simulink library "SigiLib"  (R2025b)
settings: Solver=VariableStepAuto  StartTime=0.0  StopTime=10.0  RelTol=1e-3
undefined symbols (not defined in the file): fractalcoef, X, Y, Z
libraries: sm_lib x47, nesl_utility x13, simulink x9, fl_lib x6, raspberrypiCommlib x5, $bdroot x4, ee_lib x3, mspsensorlib x1, slpidlib x1
(part 1 of 2)
settings Model: Creator=vlenzi  LastModifiedBy=resjoehr
settings RTWCC: GPUComputeCapability=3.5

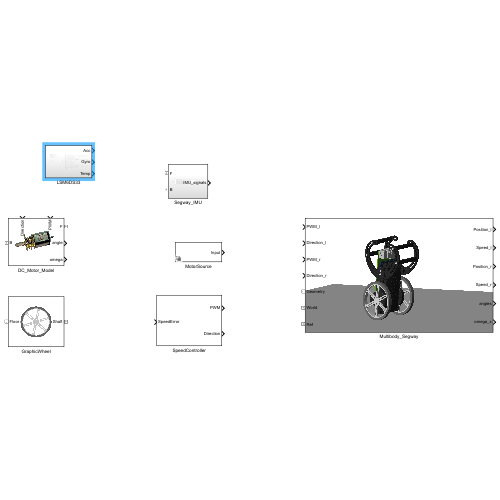
[thumbnail: Simulink's stored preview of the top-level diagram]
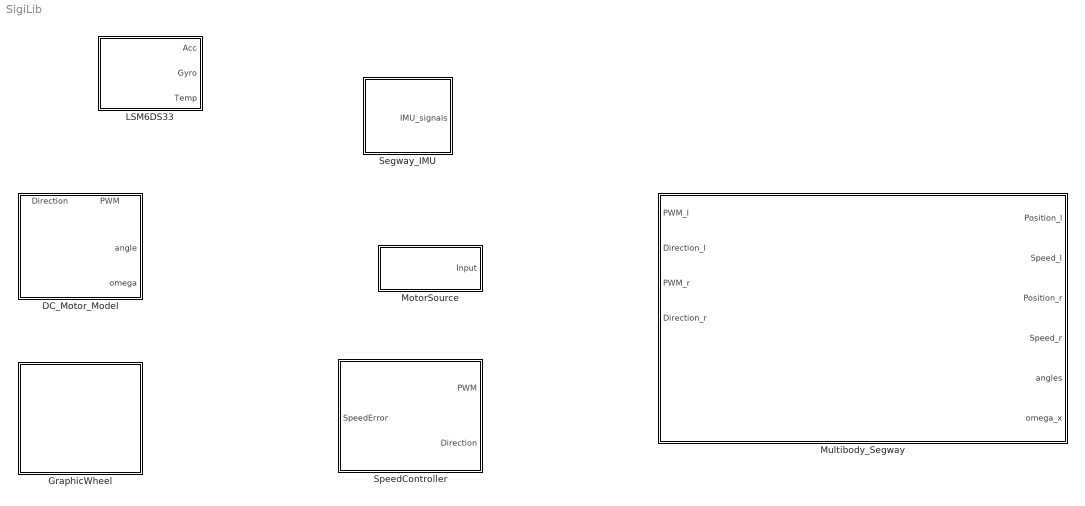
== system SigiLib ==
  DC_Motor_Model : Subsystem  mask{arm_induct=0, nlspeed=0, stall_T=0, rotor_I=0, rotor_damp=0, gear_ratio=0}
      mask prompts: arm_induct "Arm Inductance"; nlspeed "No Load Speed"; stall_T "Stall Torque"; rotor_I "Rotor Inertia"; rotor_damp "Rotor Damping"; gear_ratio "Gear Ratio (external gear box)"
      settings: PortSchema="{\"entries\":[{\"content\":{\"sides\":[{\"content\":{\"connectorIds\":[\"LConn1\"]},\"type\":\"ConnectorPlacement.EquallySpacedRectSide\",\"uuid\":\"0f359635-e508-4ae0-888d-e7a4bdac0ad6\"},{\"content\":{\"connectorIds\":[\"RConn1\",\"Out1\",\"Out2\"],\"side\":\"RIGHT\"},\"type\":\"ConnectorPlacement.EquallySpacedRectSide\",\"uuid\":\"bdc1407e-b686-4053-bd54-ae80f62d25cc\"},{\"content\":{\"connectorIds\":[\"In1\",\"In2\"],\"side\":\"TOP\"},\"type\":\"ConnectorPlacement.EquallySpacedRectSide\",\"uuid\":\"c3ebbcbf-819a-4495-8528-c62fc3c649d7\"}]},\"type\":\"ConnectorPlacement.EquallySpacedConnector\",\"uuid\":\"e7614881-2b96-4b82-8f72-d1d459cee471\"}],\"packageUris\":[\"http://schema.mathworks.com/mf0/Connector/R2020b\"],\"version\":\"1.0\"}"
      mask DialogControl Control2 Prompt: Motor parameters:
      mask DialogControl Control1 Prompt: Please specify the motor parameters. Please note, they can typically be found in the specsheet.
      mask Display: image('DC_motor.jpg');
  GraphicWheel : Subsystem
      mask Display: image('wheel.jpg', [15,15,15,15,100,100]);
  LSM6DS33 : Subsystem
  MotorSource : Subsystem  Variant=on  VariantControlMode=label  LabelModeActiveChoice=Square  mask{amp=0}
      mask prompts: amp "Amplitude"
  Multibody_Segway : Subsystem  mask{Parameter3=0, Parameter2=0}
      mask prompts: Parameter3 "Motor right"; Parameter2 "Motor left"
      mask DialogControl Container1 Prompt: Description
      mask DialogControl Control1 Prompt: This block implements the physics of the Segway using Simscape Multibody
      mask DialogControl Container2 Prompt: Parameters
      mask Display: image('whole_sigi.jpg');
  Segway_IMU : Subsystem
  SpeedController : Subsystem  mask{p_gain=0, i_gain=0, d_gain=0, n_filter=0, direction=0}
      mask prompts: p_gain "P-Gain"; i_gain "I-Gain"; d_gain "D-Gain"; n_filter "Filter"

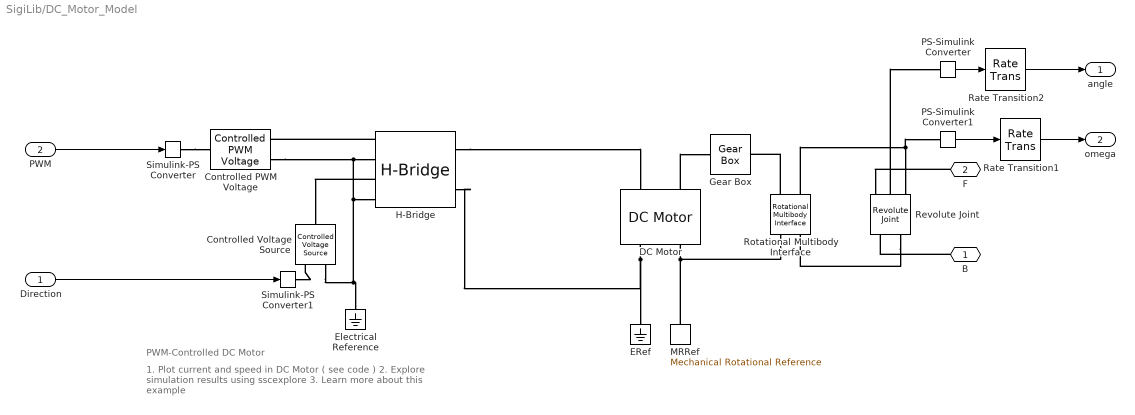
== system SigiLib/DC_Motor_Model ==
  note: PWM-Controlled DC Motor
  note: 1. Plot current and speed in DC Motor ( see code )
      | 2. Explore simulation results using sscexplore
      | 3. Learn more about this example
  Direction : Inport
  PWM : Inport  Port=2
  Controlled PWM Voltage : ee_lib/Integrated Circuits/Controlled PWM Voltage  F=1000 Hz  TD=0 s  pulse_width_offset=0 s  pulse_min=0 s  pwm_or_av=ee.enum.pwm_or_av.averaged  event_type=1  sample_time=5e-6 s  Vmin=0 V  Vmax=5 V  Vm=5 V  u_min=0  u_max=255
      settings: InternalSimscapePortConfiguration="{\"Bottom\":[],\"Left\":[{\"id\":\"u\",\"label\":\"u\",\"type\":\"input\"}],\"Right\":[{\"id\":\"p2\",\"label\":\"PWM\",\"type\":\"foundation.electrical.electrical\"},{\"id\":\"n2\",\"label\":\"REF\",\"type\":\"foundation.electrical.electrical\"}],\"Top\":[]}"
  Controlled Voltage Source : fl_lib/Electrical/Electrical Sources/Controlled Voltage Source
  DC Motor : ee_lib/Electromechanical/Brushed Motors/DC Motor  field_option=ee.enum.field_option.pm  Rf=100 Ohm  Lf=1 H  Laf=0.15 H  If0=0 A  parameterization=ee.enum.dcparam_option.torque_speed  Ra=3.38 Ohm  La=arm_induct H  emf_or_torque=ee.enum.emf_or_torque.kv  Kv=0.029 V/(rad/s)  Ki=6.876e-04 N*m/A  T_stall=stall_T N*m  w_max=nlspeed rpm  w_rated=2500 rpm  P_rated=10 W  V_rated=6 V  lam_param=ee.enum.lam_param.damping  i_noload=0 A  V_i_noload=1.5 V  J=rotor_I kg*m^2  lam=rotor_damp N*m/(rad/s)  speed0=0 rpm  alpha=3.93e-3 1/K  Tmeas=25 degC  thermal_mass=100 J/K  initial_temperature=25 degC
  ERef : fl_lib/Electrical/Electrical Elements/Electrical Reference
  Electrical Reference : fl_lib/Electrical/Electrical Elements/Electrical Reference
  Gear Box : fl_lib/Mechanical/Mechanisms/Gear Box  ratio=gear_ratio  t_in_specify=off  t_in_priority=None  t_in=0 N*m  t_in_nominal_specify=off  t_in_nominal_value=1  t_in_nominal_unit=N*m  t_out_specify=off  t_out_priority=None  t_out=0 N*m  t_out_nominal_specify=off  t_out_nominal_value=1  t_out_nominal_unit=N*m
  H-Bridge : ee_lib/Semiconductors & Converters/Converters/H-Bridge  supply_ports=ee.enum.supply_ports.hidesupply  pwm_or_av=ee.enum.pwm_or_av.averaged  regenerative_braking_mode=ee.enum.converters.regenerative_braking_mode.always_enabled  discontinuous=ee.enum.current_profile.continuous  freewheeling_mode=ee.enum.converters.freewheeling_mode.one_switch_one_diode  Rload=3.38+0.1 Ohm  Lload=1e-5 H  F=4 kHz  Venable=2.5 V  Vmax=5 V  Vreverse=.5 V  Vbrake=2.5 V  Vm=5 V  Ron=0.1 Ohm  Don=0.1 Ohm  Goff=1e-6 S  Tmeas=298.15 K  Ron2=0.1 Ohm  Don2=0.05 Ohm  Tmeas2=398.15 K  thermal_mass=100 J/K  initial_temperature=298.15 K
  MRRef : fl_lib/Mechanical/Rotational Elements/Mechanical Rotational Reference
  PS-Simulink Converter : nesl_utility/PS-Simulink Converter  PhysicalDomain=network_engine_domain  SubClassName=ps_output  LeftPortType=input  RightPortType=output  PseudoPeriodic=off  Frequencies=[]  VectorFormat=inherit  Unit=inherit  AffineConversion=off
  PS-Simulink Converter1 : nesl_utility/PS-Simulink Converter  PhysicalDomain=network_engine_domain  SubClassName=ps_output  LeftPortType=input  RightPortType=output  PseudoPeriodic=off  Frequencies=[]  VectorFormat=inherit  Unit=inherit  AffineConversion=off
  Rate Transition1 : RateTransition  OutPortSampleTime=0.01
  Rate Transition2 : RateTransition  OutPortSampleTime=0.01
  Revolute Joint : sm_lib/Joints/Revolute Joint  JointMode=Normal  CompositeWrenchDir=FollowerOnBase  CompositeWrenchFrame=BaseFrame  SenseConstraintForce=off  SenseConstraintTorque=off  SenseTotalForce=off  SenseTotalTorque=off  PositionTargetSpecify=off  PositionTargetPriority=High  PositionTargetValue=0  PositionTargetValueUnits=deg  VelocityTargetSpecify=off  VelocityTargetPriority=High  VelocityTargetValue=0  VelocityTargetValueUnits=deg/s  EquilibriumPosition=0  EquilibriumPositionUnits=deg  SpringStiffness=0  SpringStiffnessUnits=N*m/deg  DampingCoefficient=0  DampingCoefficientUnits=N*m/(deg/s)  LowerLimitSpecify=off  LowerLimitBound=-90  LowerLimitBoundUnits=deg  LowerLimitStiffness=1e4  LowerLimitStiffnessUnits=N*m/deg  LowerLimitDamping=10  LowerLimitDampingUnits=N*m/(deg/s)  LowerLimitTransitionRegionWidth=0.1  LowerLimitTransitionRegionWidthUnits=deg  UpperLimitSpecify=off  UpperLimitBound=90  UpperLimitBoundUnits=deg  UpperLimitStiffness=1e4  UpperLimitStiffnessUnits=N*m/deg  UpperLimitDamping=10  UpperLimitDampingUnits=N*m/(deg/s)  UpperLimitTransitionRegionWidth=0.1  UpperLimitTransitionRegionWidthUnits=deg  TorqueActuationMode=InputTorque  MotionActuationMode=ComputedMotion  SensePosition=on  SenseVelocity=on  SenseAcceleration=off  SenseTorqueForce=off  SenseLowerLimitTorqueForce=off  SenseUpperLimitTorqueForce=off
  Rotational Multibody Interface : fl_lib/Mechanical/Multibody Interfaces/Rotational Multibody Interface
  Simulink-PS Converter : nesl_utility/Simulink-PS Converter  PhysicalDomain=network_engine_domain  SubClassName=ps_input  LeftPortType=input  RightPortType=output  PseudoPeriodic=off  Frequencies=[]  NoiseDistribution=none  NoiseParameters=[]  Unit=1  AffineConversion=off  FilteringAndDerivatives=provide  SimscapeFilterOrder=1  InputFilterTimeConstant=0.001  UdotUserProvided=0
  Simulink-PS Converter1 : nesl_utility/Simulink-PS Converter  PhysicalDomain=network_engine_domain  SubClassName=ps_input  LeftPortType=input  RightPortType=output  PseudoPeriodic=off  Frequencies=[]  NoiseDistribution=none  NoiseParameters=[]  Unit=1  AffineConversion=off  FilteringAndDerivatives=provide  SimscapeFilterOrder=1  InputFilterTimeConstant=0.001  UdotUserProvided=0
  B : PMIOPort  Side=Left
  F : PMIOPort  Port=2  Side=Right
  angle : Outport
  omega : Outport  Port=2
  wires:
  PWM/1 -> Simulink-PS Converter/1
  Direction/1 -> Simulink-PS Converter1/1
  PS-Simulink Converter1/1 -> Rate Transition1/1
  PS-Simulink Converter/1 -> Rate Transition2/1
  Rate Transition2/1 -> angle/1
  Rate Transition1/1 -> omega/1
  connections:
  H-Bridge/RConn1 -- DC Motor/LConn1
  H-Bridge/LConn3 -- Controlled Voltage Source/LConn1
  Controlled Voltage Source/RConn2 -- Electrical Reference/LConn1 -- H-Bridge/LConn4 -- H-Bridge/LConn2 -- Controlled PWM Voltage/RConn2
  DC Motor/LConn2 -- Gear Box/LConn1
  MRRef/LConn1 -- Rotational Multibody Interface/LConn2 -- DC Motor/RConn2
  DC Motor/RConn1 -- ERef/LConn1 -- H-Bridge/RConn2
  H-Bridge/LConn1 -- Controlled PWM Voltage/RConn1
  Simulink-PS Converter/RConn1 -- Controlled PWM Voltage/LConn1
  Simulink-PS Converter1/RConn1 -- Controlled Voltage Source/RConn1
  Rotational Multibody Interface/RConn1 -- Revolute Joint/RConn3 -- PS-Simulink Converter1/LConn1
  Revolute Joint/LConn2 -- Rotational Multibody Interface/LConn1
  F/RConn1 -- Revolute Joint/RConn1
  B/RConn1 -- Revolute Joint/LConn1
  Rotational Multibody Interface/RConn2 -- Gear Box/RConn1
  Revolute Joint/RConn2 -- PS-Simulink Converter/LConn1

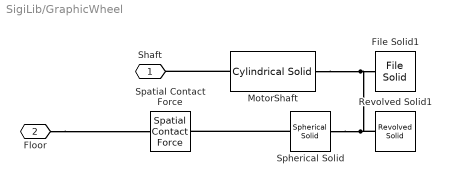
== system SigiLib/GraphicWheel ==
  File Solid1 : sm_lib/Body Elements/File Solid  ExtGeomFileName=Wheel.stl  UnitType=Custom  ExtGeomFileUnits=m  StepReaderType=HEX  ExportConvexHullGeometry=off  InertiaType=CalculateFromGeometry  BasedOnType=Density  Density=2000  DensityUnits=kg/m^3  Mass=1  MassUnits=kg  CenterOfMass=[0 0 0]  CenterOfMassUnits=m  MomentsOfInertia=[1 1 1]  MomentsOfInertiaUnits=kg*m^2  ProductsOfInertia=[0 0 0]  ProductsOfInertiaUnits=kg*m^2  GraphicType=FromGeometry  MarkerShape=Sphere  MarkerSize=10  GraphicVisPropType=SimpleVisualProperties  GraphicDiffuseColor=[1.0 1.0 1.0]  GraphicOpacity=1.0  GraphicSpecularColor=[0.5 0.5 0.5 1.0]  GraphicAmbientColor=[0.15 0.15 0.15 1.0]  GraphicEmissiveColor=[0.0 0.0 0.0 1.0]  GraphicShininess=75  DoExposeReferenceFrame=on  SerializedFrames=<Frames/>
  MotorShaft : sm_lib/Body Elements/Cylindrical Solid  CylinderRadius=1  CylinderRadiusUnits=mm  CylinderLength=10  CylinderLengthUnits=mm  ExportEntireGeometry=off  InertiaType=CalculateFromGeometry  BasedOnType=Density  Density=1000  DensityUnits=kg/m^3  Mass=1  MassUnits=kg  CenterOfMass=[0 0 0]  CenterOfMassUnits=m  MomentsOfInertia=[1 1 1]  MomentsOfInertiaUnits=kg*m^2  ProductsOfInertia=[0 0 0]  ProductsOfInertiaUnits=kg*m^2  GraphicType=FromGeometry  MarkerShape=Sphere  MarkerSize=10  GraphicVisPropType=SimpleVisualProperties  GraphicDiffuseColor=[0.5 0.5 0.5]  GraphicOpacity=1.0  GraphicSpecularColor=[0.5 0.5 0.5 1.0]  GraphicAmbientColor=[0.15 0.15 0.15 1.0]  GraphicEmissiveColor=[0.0 0.0 0.0 1.0]  GraphicShininess=75  DoExposeReferenceFrame=off  SerializedFrames=<Frames><Frame><Id>Frame1</Id><Value><Name>Bottom</Name><Origin><Source>GeometricFeature</Source><FeatureName>bottom surface</FeatureName></Origin><PrimaryAxis><DefinedDirection>+Z</DefinedDirection><Source>ReferenceFrame</Source><SourceDirection>+Z</SourceDirection><FeatureName></FeatureName></PrimaryAxis><SecondaryAxis><DefinedDirection>+X</DefinedDirection><Source>ReferenceFrame</Source><SourceDirection>+X</SourceDirection><FeatureName></FeatureName></SecondaryAxis></Value></Frame><Frame><Id>Frame2</Id><Value><Name>Top</Name><Origin><Source>GeometricFeature</Source><FeatureName>top surface</FeatureName></Origin><PrimaryAxis><DefinedDirection>+Z</DefinedDirection><Source>ReferenceFrame</Source><SourceDirection>+Z</SourceDirection><FeatureName></FeatureName></PrimaryAxis><SecondaryAxis><DefinedDirection>+X</DefinedDirection><Source>ReferenceFrame</Source><SourceDirection>+X</SourceDirection><FeatureName></FeatureName></SecondaryAxis></Value></Frame></Frames>
  Revolved Solid1 : sm_lib/Body Elements/Revolved Solid  RevolutionCrossSection=[3.5 0.5; 3.5 -0.5; 4 -0.5; 4 0.5]  RevolutionCrossSectionUnits=cm  RevolutionExtent=Full  RevolutionAngle=180  RevolutionAngleUnits=deg  ExportConvexHullGeometry=off  InertiaType=CalculateFromGeometry  BasedOnType=Density  Density=0  DensityUnits=kg/m^3  Mass=1  MassUnits=kg  CenterOfMass=[0 0 0]  CenterOfMassUnits=m  MomentsOfInertia=[1 1 1]  MomentsOfInertiaUnits=kg*m^2  ProductsOfInertia=[0 0 0]  ProductsOfInertiaUnits=kg*m^2  GraphicType=FromGeometry  MarkerShape=Sphere  MarkerSize=10  GraphicVisPropType=SimpleVisualProperties  GraphicDiffuseColor=[0.5 0.5 0.5]  GraphicOpacity=1.0  GraphicSpecularColor=[0.5 0.5 0.5 1.0]  GraphicAmbientColor=[0.15 0.15 0.15 1.0]  GraphicEmissiveColor=[0.0 0.0 0.0 1.0]  GraphicShininess=75  DoExposeReferenceFrame=on  SerializedFrames=<Frames/>
  Spatial Contact Force : sm_lib/Forces and Torques/Spatial Contact Force  SenseSeparationDistance=off  NormalForceType=SmoothSpringDamper  NormalStiffness=1e6  NormalStiffnessUnits=N/m  NormalDamping=1e3  NormalDampingUnits=N/(m/s)  NormalTransitionRegionWidth=1e-4  NormalTransitionRegionWidthUnits=m  FrictionType=SmoothStickSlip  CoefficientOfStaticFriction=1  CoefficientOfDynamicFriction=0.7  FrictionalCriticalVelocity=0.001  FrictionalCriticalVelocityUnits=m/s  SenseContactSignal=off  SensePenetrationDepth=off  SenseNormalVelocity=off  SenseTangentialVelocity=off  SensingForceTorqueDirection=BaseOnFollower  SensingForceTorqueResolutionFrame=ContactFrame  SenseNormalForce=off  SenseNormalForceMagnitude=off  SenseNormalTorque=off  SenseFrictionalForce=off  SenseFrictionalForceMagnitude=off  SenseFrictionalTorque=off  SenseTotalForce=off  SenseTotalTorque=off  SenseContactBaseRotation=off  SenseContactBaseTranslation=off  SenseContactFollowerRotation=off  SenseContactFollowerTranslation=off  ZeroCrossDetectContactStartAndEnd=off
  Spherical Solid : sm_lib/Body Elements/Spherical Solid  SphereRadius=4.05  SphereRadiusUnits=cm  ExportEntireGeometry=on  InertiaType=CalculateFromGeometry  BasedOnType=Density  Density=0  DensityUnits=kg/m^3  Mass=1  MassUnits=kg  CenterOfMass=[0 0 0]  CenterOfMassUnits=m  MomentsOfInertia=[1 1 1]  MomentsOfInertiaUnits=kg*m^2  ProductsOfInertia=[0 0 0]  ProductsOfInertiaUnits=kg*m^2  GraphicType=FromGeometry  MarkerShape=Sphere  MarkerSize=10  GraphicVisPropType=SimpleVisualProperties  GraphicDiffuseColor=[0.6 0 0]  GraphicOpacity=0.1  GraphicSpecularColor=[0.5 0.5 0.5 1.0]  GraphicAmbientColor=[0.15 0.15 0.15 1.0]  GraphicEmissiveColor=[0.0 0.0 0.0 1.0]  GraphicShininess=75  DoExposeReferenceFrame=on  SerializedFrames=<Frames/>
  Shaft : PMIOPort  Side=Right
  Floor : PMIOPort  Port=2  Side=Left
  connections:
  File Solid1/RConn1 -- MotorShaft/RConn1 -- Spherical Solid/RConn1 -- Revolved Solid1/RConn1
  Floor/RConn1 -- Spatial Contact Force/RConn1
  MotorShaft/LConn1 -- Shaft/RConn1
  Spherical Solid/LConn1 -- Spatial Contact Force/LConn1

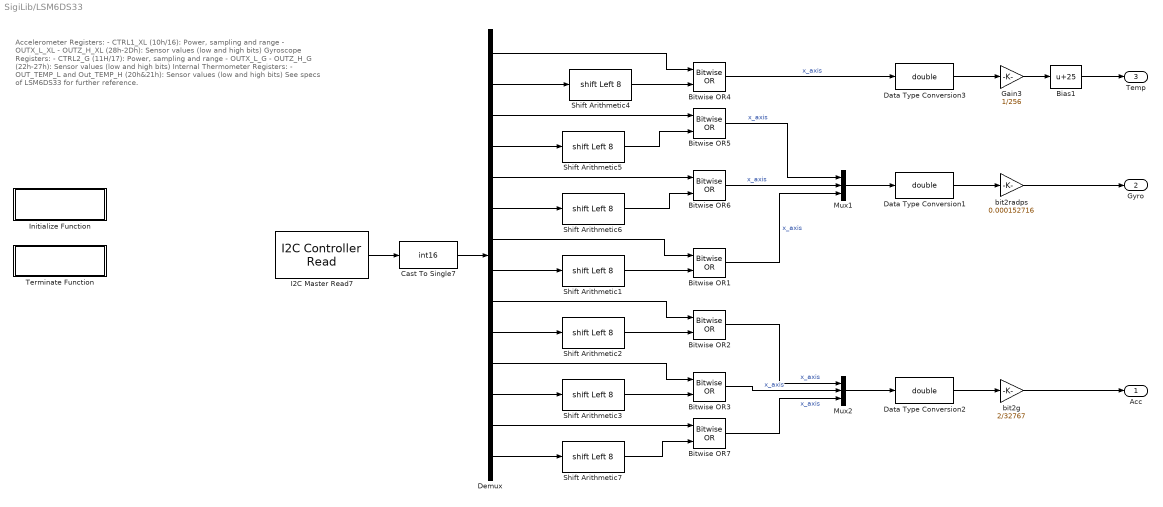
== system SigiLib/LSM6DS33 ==
  note: Accelerometer Registers:
      | - CTRL1_XL (10h/16): Power, sampling and range
      | - OUTX_L_XL - OUTZ_H_XL (28h-2Dh): Sensor values (low and high bits)
      |
      | Gyroscope Registers:
      | - CTRL2_G (11H/17): Power, sampling and range
      | - OUTX_L_G - OUTZ_H_G (22h-27h): Sensor values (low and high bits)
      |
      | Internal Thermometer Registers:
      | - OUT_TEMP_L and Out_TEMP_H (20h&21h): Sensor values (low and high bits)
      |
      | See specs of LSM6DS33 for further reference.
  Bias1 : Bias  Bias=25  SaturateOnIntegerOverflow=off
  Bitwise OR{1..7} (7 alike) : simulink/Logic and Bit Operations/Bitwise Operator  logicop=OR  UseBitMask=off  NumInputPorts=2  BitMask=bin2dec('11011001')  BitMaskRealWorld=Stored Integer
  Cast To Single7 : DataTypeConversion  OutDataTypeStr=int16  SaturateOnIntegerOverflow=off  RndMeth=Floor
  Data Type Conversion1 : DataTypeConversion  OutDataTypeStr=double  SaturateOnIntegerOverflow=off  RndMeth=Floor
  Data Type Conversion2 : DataTypeConversion  OutDataTypeStr=double  SaturateOnIntegerOverflow=off  RndMeth=Floor
  Data Type Conversion3 : DataTypeConversion  OutDataTypeStr=double  SaturateOnIntegerOverflow=off  RndMeth=Floor
  Demux : Demux  Outputs=14
  Gain3 : Gain  Gain=1/256
  I2C Master Read7 : raspberrypiCommlib/I2C Controller Read  BoardProperty=Pi 3 Model B+  I2CModule=1  Mode=Master  SlaveAddress=107  SlaveByteOrder=BigEndian  Direction=Receiver  RegisterAddressMode=on  RegisterAddress=hex2dec('20')  SlaveDataType=uint8  DataLength=14  NoAck=off  RepeatedStart=off  OutputStatus=off  SampleTime=0.01
  Initialize Function : Subsystem  TreatAsAtomicUnit=on
  Mux1 : Mux  Inputs=3
  Mux2 : Mux  Inputs=3
  Shift Arithmetic{1..7} (7 alike) : ArithShift  BitShiftNumber=8  BitShiftDirection=Left
  Terminate Function : Subsystem  TreatAsAtomicUnit=on
  bit2g : Gain  Gain=2/32767
  bit2radps : Gain  Gain=0.000152716
  Acc : Outport  Unit=g
  Gyro : Outport  Port=2  Unit=rad/s
  Temp : Outport  Port=3
  wires:
  Cast To Single7/1 -> Demux/1
  Shift Arithmetic4/1 -> Bitwise OR4/2
  Bitwise OR4/1 -> Data Type Conversion3/1  "x_axis"
  Shift Arithmetic6/1 -> Bitwise OR6/2
  Demux/1 -> Bitwise OR4/1
  Mux1/1 -> Data Type Conversion1/1
  Demux/5 -> Bitwise OR6/1
  Demux/6 -> Shift Arithmetic6/1
  I2C Master Read7/1 -> Cast To Single7/1
  Bitwise OR6/1 -> Mux1/2  "x_axis"
  Demux/4 -> Shift Arithmetic5/1
  Shift Arithmetic5/1 -> Bitwise OR5/2
  Demux/3 -> Bitwise OR5/1
  Demux/2 -> Shift Arithmetic4/1
  Bitwise OR5/1 -> Mux1/1  "x_axis"
  Data Type Conversion1/1 -> bit2radps/1
  Shift Arithmetic3/1 -> Bitwise OR3/2
  Bitwise OR3/1 -> Mux2/2  "x_axis"
  Bitwise OR1/1 -> Mux1/3  "x_axis"
  Shift Arithmetic1/1 -> Bitwise OR1/2
  Demux/7 -> Bitwise OR1/1
  Mux2/1 -> Data Type Conversion2/1
  Bitwise OR2/1 -> Mux2/1  "x_axis"
  Shift Arithmetic2/1 -> Bitwise OR2/2
  Demux/9 -> Bitwise OR2/1
  Demux/10 -> Shift Arithmetic2/1
  Demux/8 -> Shift Arithmetic1/1
  Demux/11 -> Bitwise OR3/1
  Demux/12 -> Shift Arithmetic3/1
  Demux/13 -> Bitwise OR7/1
  Shift Arithmetic7/1 -> Bitwise OR7/2
  Demux/14 -> Shift Arithmetic7/1
  Bitwise OR7/1 -> Mux2/3  "x_axis"
  Data Type Conversion2/1 -> bit2g/1
  Gain3/1 -> Bias1/1
  Bias1/1 -> Temp/1
  Data Type Conversion3/1 -> Gain3/1
  bit2g/1 -> Acc/1
  bit2radps/1 -> Gyro/1

== system SigiLib/MotorSource ==
  note: 1) Add Subsystem or Model blocks as valid variant choices.
      | 2) You cannot connect blocks at this level. At simulation, connectivity is automatically
      | determined, based on the active variant and port name matching.
  Subsystem : Subsystem  VariantControl=Custom
  Subsystem1 : Subsystem  VariantControl=Square
  Subsystem2 : Subsystem  VariantControl=Ramp
  Input : Outport

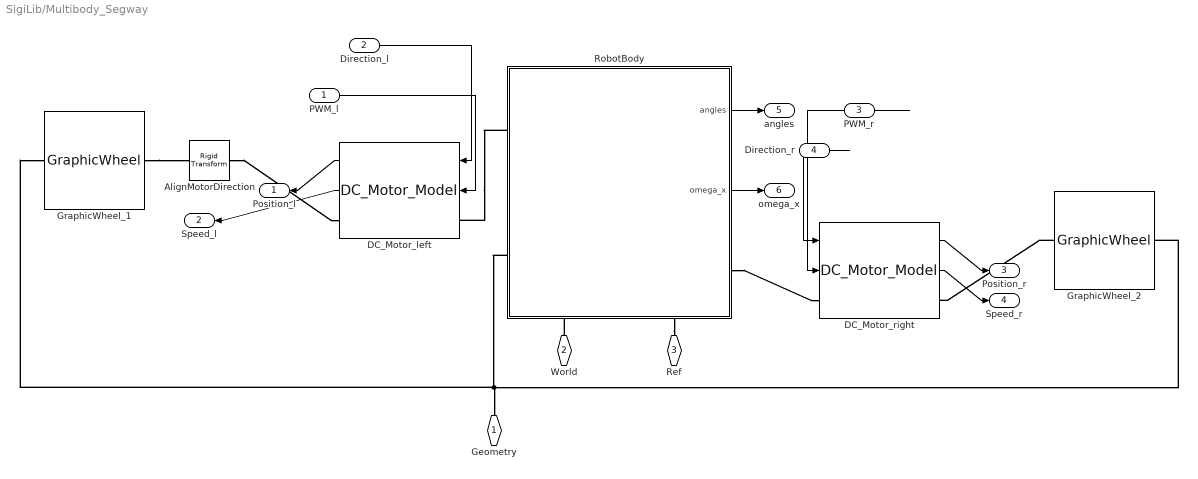
== system SigiLib/Multibody_Segway ==
  PWM_l : Inport
  Direction_l : Inport  Port=2
  PWM_r : Inport  Port=3
  Direction_r : Inport  Port=4
  AlignMotorDirection : sm_lib/Frames and Transforms/Rigid Transform  RotationMethod=StandardAxis  FollAlignAxisA=+Z  BaseAlignAxisA=-Z  FollAlignAxisB=+Y  BaseAlignAxisB=+Z  RotationStandardAxis=+Y  RotationAngle=180  RotationAngleUnits=deg  RotationArbitraryAxis=[0 0 1]  RotationSequenceAxes=FollowerAxes  RotationSequence=XYX  RotationSequenceAngles=[0 0 0]  RotationSequenceAnglesUnits=deg  RotationMatrix=[1 0 0; 0 1 0; 0 0 1]  Quaternion=[1 0 0 0]  TranslationMethod=None  TranslationCartesianOffset=[0 0 -0.014]  TranslationCartesianOffsetUnits=m  TranslationStandardAxis=+Z  TranslationStandardOffset=0  TranslationStandardOffsetUnits=m  TranslationROffset=0  TranslationROffsetUnits=m  TranslationThetaOffset=0  TranslationThetaOffsetUnits=deg  TranslationZOffset=0  TranslationZOffsetUnits=m
  DC_Motor_left : $bdroot/DC_Motor_Model  arm_induct=motor_left.arm_induct  nlspeed=motor_left.nlspeed  stall_T=motor_left.stall_T  rotor_I=motor_left.rotor_I  rotor_damp=motor_left.rotor_damp  gear_ratio=motor_left.gear_ratio
  DC_Motor_right : $bdroot/DC_Motor_Model  arm_induct=motor_right.arm_induct  nlspeed=motor_right.nlspeed  stall_T=motor_right.stall_T  rotor_I=motor_right.rotor_I  rotor_damp=motor_right.rotor_damp  gear_ratio=motor_right.gear_ratio
  GraphicWheel_1 : $bdroot/GraphicWheel  SystemSampleTime=-1  VariantActivationTime=update diagram  EmptyChoice=off  PassThrough=off  PassThroughVariantControl=(default)  EmptyChoiceVariantControl=(default)  AllowFlexibleInterface=on  Latency=0  AutoFrameSizeCalculation=off
      link override Spherical Solid: GraphicOpacity=0.4
  GraphicWheel_2 : $bdroot/GraphicWheel  SystemSampleTime=-1  VariantActivationTime=update diagram  EmptyChoice=off  PassThrough=off  PassThroughVariantControl=(default)  EmptyChoiceVariantControl=(default)  AllowFlexibleInterface=on  Latency=0  AutoFrameSizeCalculation=off
  RobotBody : Subsystem
      settings: PortSchema="{\"entries\":[{\"content\":{\"sides\":[{\"content\":{\"connectorIds\":[\"LConn1\",\"LConn2\"]},\"type\":\"ConnectorPlacement.EquallySpacedRectSide\",\"uuid\":\"3f35a83b-acf9-4542-85ca-c3be7738438d\"},{\"content\":{\"connectorIds\":[\"Out1\",\"Out2\",\"RConn1\"],\"side\":\"RIGHT\"},\"type\":\"ConnectorPlacement.EquallySpacedRectSide\",\"uuid\":\"c08ff41f-e4b1-40fb-853d-24ced0702649\"},{\"content\":{\"side\":\"TOP\"},\"type\":\"ConnectorPlacement.EquallySpacedRectSide\",\"uuid\":\"d298c9e2-1711-4257-8e5b-24fb1711ca30\"},{\"content\":{\"connectorIds\":[\"RConn2\",\"RConn3\"],\"side\":\"BOTTOM\"},\"type\":\"ConnectorPlacement.EquallySpacedRectSide\",\"uuid\":\"0a2d3d52-b6dd-493e-8124-2dc32b2e7700\"}]},\"type\":\"ConnectorPlacement.EquallySpacedConnector\",\"uuid\":\"2a993940-985c-47f0-a186-f410faa28ad3\"}],\"packageUris\":[\"http://schema.mathworks.com/mf0/Connector/R2020b\"],\"version\":\"1.0\"}"
      mask Display: image('sigi_body.jpg');
  Geometry : PMIOPort  Side=Left
  World : PMIOPort  Port=2  Side=Left
  Ref : PMIOPort  Port=3  Side=Left
  Position_l : Outport
  Speed_l : Outport  Port=2
  Position_r : Outport  Port=3
  Speed_r : Outport  Port=4
  angles : Outport  Port=5
  omega_x : Outport  Port=6
  wires:
  DC_Motor_right/2 -> Speed_r/1
  DC_Motor_left/2 -> Speed_l/1
  DC_Motor_right/1 -> Position_r/1
  PWM_r/1 -> DC_Motor_right/2
  Direction_r/1 -> DC_Motor_right/1
  RobotBody/2(omega_x) -> omega_x/1
  RobotBody/1(angles) -> angles/1
  DC_Motor_left/1 -> Position_l/1
  Direction_l/1 -> DC_Motor_left/1
  PWM_l/1 -> DC_Motor_left/2
  connections:
  RobotBody/LConn1 -- DC_Motor_left/LConn1
  AlignMotorDirection/LConn1 -- DC_Motor_left/RConn1
  RobotBody/RConn1 -- DC_Motor_right/LConn1
  GraphicWheel_1/RConn1 -- AlignMotorDirection/RConn1
  RobotBody/LConn2 -- GraphicWheel_1/LConn1 -- GraphicWheel_2/LConn1 -- Geometry/RConn1
  World/RConn1 -- RobotBody/RConn2
  GraphicWheel_2/RConn1 -- DC_Motor_right/RConn1
  RobotBody/RConn3 -- Ref/RConn1

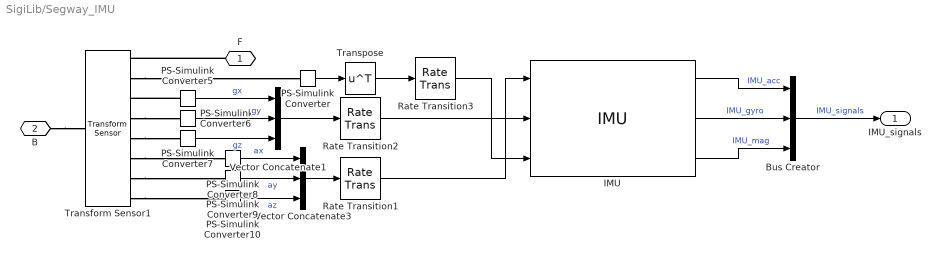
== system SigiLib/Segway_IMU ==
  Bus Creator : BusCreator  Inputs=3  OutDataTypeStr=Bus: IMU_signals
      settings: InheritFromInputs=off
  IMU : mspsensorlib/IMU  DispRefFrame=NED  TemperaturePort=off  Temperature=25  MagneticFieldPort=off  MagneticFieldNED=[ 27.5550, -2.4169, -16.0849 ]  MagneticFieldENU=[ -2.4169, 27.5550, 16.0849 ]  SeedDouble=67  SimulateUsing=Interpreted execution  AccelParamsMeasurementRange=19.62  AccelParamsResolution=5.9841e-4  AccelParamsConstantBias=[ 0, 0, 0 ]  AccelParamsAxesMisalignment=[ 100, 0, 0; 0, 100, 0; 0, 0, 100 ]  AccelParamsNoiseDensity=[ 0.1213e-3, 0.1072e-3, 0.2141e-3 ]  AccelParamsBiasInstability=[ 0.0402e-3, 0.0923e-3, 0.137e-3 ]  AccelParamsBiasInstabilityNumerator=fractalcoef().Numerator  AccelParamsBiasInstabilityDenominator=fractalcoef().Denominator  AccelParamsRandomWalk=[ 0.0399e-4, 0.1093e-4, 0.3611e-4 ]  AccelParamsNoiseType=double-sided  AccelParamsTemperatureBias=[ 0, 0, 0 ]  AccelParamsTemperatureScaleFactor=[ 0, 0, 0 ]  GyroParamsMeasurementRange=245  GyroParamsResolution=0.00875  GyroParamsConstantBias=[ 0.0527, -0.1277, -0.0283 ]  GyroParamsAxesMisalignment=[ 100, 0, 0; 0, 100, 0; 0, 0, 100 ]  GyroParamsAccelerationBias=[ 0, 0, 0 ]  GyroParamsNoiseDensity=[ 0.0034, 0.0046, 0.0016 ]  GyroParamsBiasInstability=[ 0.0006069, 0.0009649, 0.0004479 ]  GyroParamsBiasInstabilityNumerator=fractalcoef().Numerator  GyroParamsBiasInstabilityDenominator=fractalcoef().Denominator  GyroParamsRandomWalk=[ 0.00005272, 0.00007008, 0.00005776 ]  GyroParamsNoiseType=double-sided  GyroParamsTemperatureBias=[ 0, 0, 0 ]  GyroParamsTemperatureScaleFactor=[ 0, 0, 0 ]  MagParamsMeasurementRange=Inf  MagParamsResolution=0  MagParamsConstantBias=[ 0, 0, 0 ]  MagParamsAxesMisalignment=[ 100, 0, 0; 0, 100, 0; 0, 0, 100 ]  MagParamsNoiseDensity=[ 0, 0, 0 ]  MagParamsBiasInstability=[ 0, 0, 0 ]  MagParamsBiasInstabilityNumerator=fractalcoef().Numerator  MagParamsBiasInstabilityDenominator=fractalcoef().Denominator  MagParamsRandomWalk=[ 0, 0, 0 ]  MagParamsNoiseType=double-sided  MagParamsTemperatureBias=[ 0, 0, 0 ]  MagParamsTemperatureScaleFactor=[ 0, 0, 0 ]
  PS-Simulink Converter{,5..10} (7 alike) : nesl_utility/PS-Simulink Converter  PhysicalDomain=network_engine_domain  SubClassName=ps_output  LeftPortType=input  RightPortType=output  PseudoPeriodic=off  Frequencies=[]  VectorFormat=inherit  Unit=inherit  AffineConversion=off
  Rate Transition1 : RateTransition  OutPortSampleTime=0.01
  Rate Transition2 : RateTransition  OutPortSampleTime=0.01
  Rate Transition3 : RateTransition  OutPortSampleTime=0.01
  Transform Sensor1 : sm_lib/Frames and Transforms/Transform Sensor  MeasurementFrame=World  RotationSequence=XYX  SenseAngle=off  SenseAxis=off  SenseQ=on  SenseR=off  SenseRotationSequence=off  SenseOmegaX=on  SenseOmegaY=on  SenseOmegaZ=on  SenseOmega=off  SenseQDot=off  SenseRDot=off  SenseRotationSequenceDot=off  SenseAlphaX=off  SenseAlphaY=off  SenseAlphaZ=off  SenseAlpha=off  SenseQDDot=off  SenseRDDot=off  SenseX=off  SenseY=off  SenseZ=off  SenseXYZ=off  SenseRad=off  SenseAzim=off  SenseDist=off  SenseInc=off  SenseXDot=off  SenseYDot=off  SenseZDot=off  SenseXYZDot=off  SenseRadDot=off  SenseAzimDot=off  SenseDistDot=off  SenseIncDot=off  SenseXDDot=on  SenseYDDot=on  SenseZDDot=on  SenseXYZDDot=off  SenseRadDDot=off  SenseAzimDDot=off  SenseDistDDot=off  SenseIncDDot=off
  Transpose : Math  Operator=transpose
  Vector Concatenate1 : Concatenate  NumInputs=3  Mode=Multidimensional array  ConcatenateDimension=2
  Vector Concatenate3 : Concatenate  NumInputs=3  Mode=Multidimensional array  ConcatenateDimension=2
  F : PMIOPort  Side=Left
  B : PMIOPort  Port=2  Side=Left
  IMU_signals : Outport
  wires:
  PS-Simulink Converter5/1 -> Vector Concatenate1/1  "gx"
  PS-Simulink Converter6/1 -> Vector Concatenate1/2  "gy"
  PS-Simulink Converter7/1 -> Vector Concatenate1/3  "gz"
  PS-Simulink Converter8/1 -> Vector Concatenate3/1  "ax"
  PS-Simulink Converter9/1 -> Vector Concatenate3/2  "ay"
  PS-Simulink Converter10/1 -> Vector Concatenate3/3  "az"
  Vector Concatenate1/1 -> Rate Transition2/1
  Vector Concatenate3/1 -> Rate Transition1/1
  PS-Simulink Converter/1 -> Transpose/1
  Transpose/1 -> Rate Transition3/1
  IMU/1 -> Bus Creator/1  "IMU_acc"
  IMU/2 -> Bus Creator/2  "IMU_gyro"
  Rate Transition1/1 -> IMU/1
  Rate Transition2/1 -> IMU/2
  Rate Transition3/1 -> IMU/3
  IMU/3 -> Bus Creator/3  "IMU_mag"
  Bus Creator/1 -> IMU_signals/1  "IMU_signals"
  connections:
  F/RConn1 -- Transform Sensor1/RConn1
  B/RConn1 -- Transform Sensor1/LConn1
  PS-Simulink Converter5/LConn1 -- Transform Sensor1/RConn3
  Transform Sensor1/RConn4 -- PS-Simulink Converter6/LConn1
  Transform Sensor1/RConn5 -- PS-Simulink Converter7/LConn1
  Transform Sensor1/RConn6 -- PS-Simulink Converter8/LConn1
  Transform Sensor1/RConn7 -- PS-Simulink Converter9/LConn1
  Transform Sensor1/RConn8 -- PS-Simulink Converter10/LConn1
  Transform Sensor1/RConn2 -- PS-Simulink Converter/LConn1

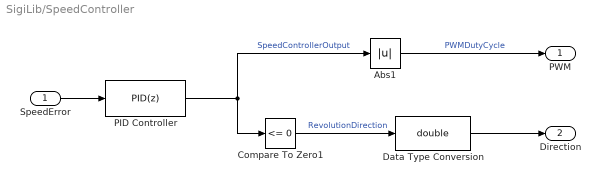
== system SigiLib/SpeedController ==
  SpeedError : Inport
  Abs1 : Abs  SaturateOnIntegerOverflow=off  OutDataTypeStr=Inherit: Inherit via internal rule
  Compare To Zero1 : simulink/Logic and Bit Operations/Compare To Zero  relop=<=  OutDataTypeStr=boolean
  Data Type Conversion : DataTypeConversion  OutDataTypeStr=double  SaturateOnIntegerOverflow=off  RndMeth=Floor
  PID Controller : slpidlib/PID Controller  Controller=PID  Form=Parallel  TimeDomain=Discrete-time  UseExternalTs=off  SampleTime=0.01  IntegratorMethod=Forward Euler  FilterMethod=Forward Euler  ControllerParametersSource=internal  P=p_gain  I=i_gain  UseKiTs=off  D=d_gain  UseExternalDerivativeSource=off  N=n_filter  UseFilter=on  TunerSelectOption=Transfer Function Based (PID Tuner App)  InitialConditionSource=internal  InitialConditionForIntegrator=0  InitialConditionForFilter=0  DifferentiatorICPrevScaledInput=0  ExternalReset=none  TrackingMode=off  Kt=1  LimitOutput=on  SatLimitsSource=internal  UpperSaturationLimit=250  LowerSaturationLimit=-250  LinearizeAsGain=on  AntiWindupMode=back-calculation  Kb=1  LimitIntegrator=off  UpperIntegratorSaturationLimit=inf  LowerIntegratorSaturationLimit=-inf  POutMin=[]  POutMax=[]  IOutMin=[]  IOutMax=[]  DOutMin=[]  DOutMax=[]  NOutMin=[]  NOutMax=[]  SumOutMin=[]  SumOutMax=[]  SaturationOutMin=[]  SaturationOutMax=[]  PParamMin=[]  PParamMax=[]  IParamMin=[]  IParamMax=[]  DParamMin=[]  DParamMax=[]  NParamMin=[]  NParamMax=[]  KbParamMin=[]  KbParamMax=[]  KtParamMin=[]  KtParamMax=[]  KbOutMin=[]  KbOutMax=[]  KtOutMin=[]  KtOutMax=[]  IntegratorOutMin=[]  IntegratorOutMax=[]  FilterOutMin=[]  FilterOutMax=[]  SumI1OutMin=[]  SumI1OutMax=[]  SumI2OutMin=[]  SumI2OutMax=[]  SumI3OutMin=[]  SumI3OutMax=[]  SumI4OutMin=[]  SumI4OutMax=[]  SumDOutMin=[]  SumDOutMax=[]  DifferentiatorOutMin=[]  DifferentiatorOutMax=[]  FilterDiffOutCoefMin=[]  FilterDiffOutCoefMax=[]  ReciprocalOutMin=[]  ReciprocalOutMax=[]  SumDenOutMin=[]  SumDenOutMax=[]  SumNumOutMin=[]  SumNumOutMax=[]  DivideOutMin=[]  DivideOutMax=[]  UdiffTsProdOutMin=[]  UdiffTsProdOutMax=[]  NTsProdOutMin=[]  NTsProdOutMax=[]  UintegralTsProdOutMin=[]  UintegralTsProdOutMax=[]  UngainTsProdOutMin=[]  UngainTsProdOutMax=[]  ClampingZeroOutDataTypeStr=Inherit: Inherit via back propagation  ClampingZeroOutMin=[]  ClampingZeroOutMax=[]  FilterDenConstantOutDataTypeStr=Inherit: Inherit via back propagation  FilterDenConstantOutMin=[]  FilterDenConstantOutMax=[]  PCopyOutDataTypeStr=Inherit: Inherit via back propagation  PCopyOutMin=[]  PCopyOutMax=[]  NCopyOutDataTypeStr=Inherit: Inherit via back propagation  NCopyOutMin=[]  NCopyOutMax=[]  IntegratorContinuousStateAttributes=''  IntegratorStateMustResolveToSignalObject=off  IntegratorRTWStateStorageClass=Auto  FilterContinuousStateAttributes=''  FilterStateMustResolveToSignalObject=off  FilterRTWStateStorageClass=Auto  ParallelPVariant=InternalParameters  IdealPVariant=Disabled  IVariant=InternalParameters  DVariant=InternalParameters  IntegratorVariant=Discrete  SatVariant=Enabled  AWVariant=BackCalculation  PCopyVariant=Disabled  TRVariant=Disabled  FdbkBlocksVariant=Forward  IdealPFdbkVariant=Disabled  SatFdbkVariant=Disabled  DerivativeFilterVariant=ForwardEulerFilter  NVariant=InternalParameters  NCopyVariant=Disabled  FilterICVariant=InternalICsFilter  IntegratorICVariant=InternalICs  ExternalResetVariant=Disabled  TRSumVariant=Passthrough  SumFdbkVariant=Disabled  SumVariant=Sum_PID  TsampFilterVariant=InternalTs  TsampNgainVariant=Passthrough  TsampIntegralVariant=Disabled_SignalSpec  ExternalSaturationOutDataTypeStr=Inherit: Same as second input  DerivativeSourceVariant=ErrorSignal  PreIntVariant=InternalPreInt
  PWM : Outport
  Direction : Outport  Port=2
  wires:
  PID Controller/1 -> Compare To Zero1/1, Abs1/1  "SpeedControllerOutput"
  Data Type Conversion/1 -> Direction/1
  Abs1/1 -> PWM/1  "PWMDutyCycle"
  SpeedError/1 -> PID Controller/1
  Compare To Zero1/1 -> Data Type Conversion/1  "RevolutionDirection"

== system SigiLib/LSM6DS33/Initialize Function ==
  note: Initiate the IMU - Setting sample rate and sensor range
  Constant : Constant  Value=64
  Constant2 : Constant  Value=64
  Data Type Conversion : DataTypeConversion  OutDataTypeStr=uint8  SaturateOnIntegerOverflow=off  RndMeth=Floor
  Data Type Conversion1 : DataTypeConversion  OutDataTypeStr=uint8  SaturateOnIntegerOverflow=off  RndMeth=Floor
  Event Listener : EventListener  DisableCoverage=on  EventName=reset
  I2C acc write : raspberrypiCommlib/I2C Controller Write  BoardProperty=Pi 3 Model B+  I2CModule=1  Mode=Master  SlaveAddress=107  SlaveByteOrder=BigEndian  Direction=Transmitter  RegisterAddressMode=on  RegisterAddress=16  SlaveDataType=uint8  DataLength=1  NoAck=off  RepeatedStart=off  OutputStatus=off
  I2C gyro write : raspberrypiCommlib/I2C Controller Write  BoardProperty=Pi 3 Model B+  I2CModule=1  Mode=Master  SlaveAddress=107  SlaveByteOrder=BigEndian  Direction=Transmitter  RegisterAddressMode=on  RegisterAddress=17  SlaveDataType=uint8  DataLength=1  NoAck=off  RepeatedStart=off  OutputStatus=off
  wires:
  Constant2/1 -> Data Type Conversion/1
  Data Type Conversion/1 -> I2C gyro write/1
  Data Type Conversion1/1 -> I2C acc write/1
  Constant/1 -> Data Type Conversion1/1

== system SigiLib/LSM6DS33/Terminate Function ==
  Constant : Constant  Value=0
  Constant2 : Constant  Value=0
  Data Type Conversion1 : DataTypeConversion  OutDataTypeStr=uint8  SaturateOnIntegerOverflow=off  RndMeth=Floor
  Data Type Conversion2 : DataTypeConversion  OutDataTypeStr=uint8  SaturateOnIntegerOverflow=off  RndMeth=Floor
  Event Listener : EventListener  DisableCoverage=on  EventType=Terminate  EventName=reset
  I2C Master Write : raspberrypiCommlib/I2C Controller Write  BoardProperty=Pi 3 Model B+  I2CModule=1  Mode=Master  SlaveAddress=107  SlaveByteOrder=BigEndian  Direction=Transmitter  RegisterAddressMode=on  RegisterAddress=17  SlaveDataType=uint8  DataLength=1  NoAck=off  RepeatedStart=off  OutputStatus=off
  I2C Master Write2 : raspberrypiCommlib/I2C Controller Write  BoardProperty=Pi 3 Model B+  I2CModule=1  Mode=Master  SlaveAddress=107  SlaveByteOrder=BigEndian  Direction=Transmitter  RegisterAddressMode=on  RegisterAddress=16  SlaveDataType=uint8  DataLength=1  NoAck=off  RepeatedStart=off  OutputStatus=off
  wires:
  Data Type Conversion1/1 -> I2C Master Write/1
  Constant/1 -> Data Type Conversion2/1
  Data Type Conversion2/1 -> I2C Master Write2/1
  Constant2/1 -> Data Type Conversion1/1

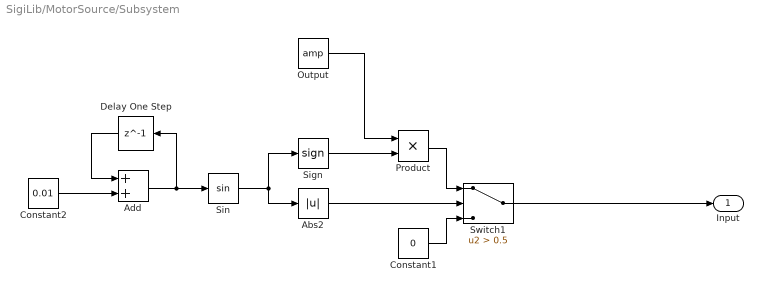
== system SigiLib/MotorSource/Subsystem ==
  Abs2 : Abs  OutDataTypeStr=single  SaturateOnIntegerOverflow=off
  Add : Sum  OutDataTypeStr=double
  Constant1 : Constant  Value=0  OutDataTypeStr=single  SampleTime=0.01
  Constant2 : Constant  Value=0.01
  Delay One Step : Delay  DelayLength=1  SampleTime=0.01
  Output : Constant  Value=amp  OutDataTypeStr=single  SampleTime=0.01
  Product : Product
  Sign : Signum
  Sin : Trigonometry  OutputSignalType=real
  Switch1 : Switch  Criteria=u2 > Threshold  Threshold=0.5  SaturateOnIntegerOverflow=off  InputSameDT=off
  Input : Outport
  wires:
  Switch1/1 -> Input/1
  Abs2/1 -> Switch1/2
  Add/1 -> Delay One Step/1, Sin/1
  Sin/1 -> Abs2/1, Sign/1
  Output/1 -> Product/1
  Product/1 -> Switch1/1
  Sign/1 -> Product/2
  Constant2/1 -> Add/2
  Delay One Step/1 -> Add/1
  Constant1/1 -> Switch1/3

== system SigiLib/MotorSource/Subsystem1 ==
  PWM_input : SignalGenerator  WaveForm=square  Amplitude=amp  Frequency=0.3
  Input : Outport
  wires:
  PWM_input/1 -> Input/1

== system SigiLib/MotorSource/Subsystem2 ==
  Ramp : simulink/Sources/Ramp  slope=amp/10  start=0  InitialOutput=0
  Input : Outport
  wires:
  Ramp/1 -> Input/1

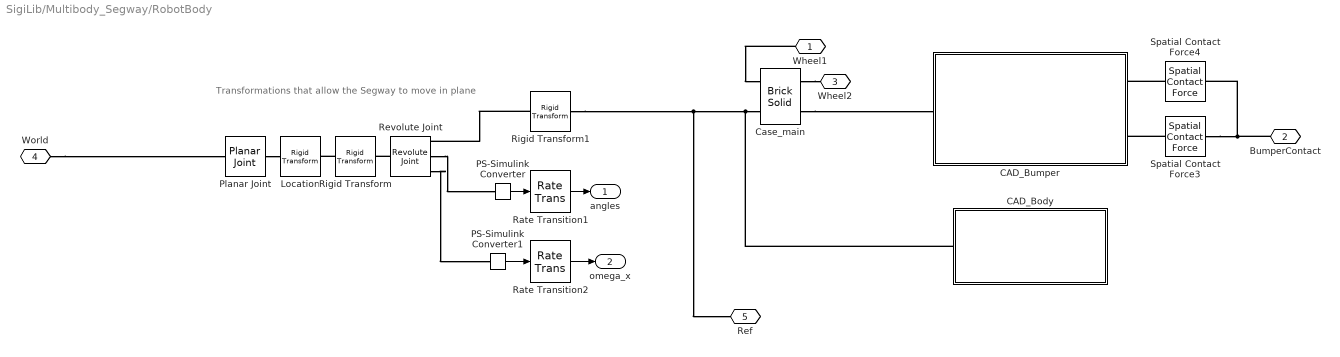
== system SigiLib/Multibody_Segway/RobotBody ==
  note: Transformations that allow the Segway to move in plane
  CAD_Body : Subsystem
  CAD_Bumper : Subsystem
  Case_main : sm_lib/Body Elements/Brick Solid  BrickDimensions=[8 5.5 2]  BrickDimensionsUnits=cm  ExportEntireGeometry=off  InertiaType=CalculateFromGeometry  BasedOnType=Density  Density=0  DensityUnits=kg/m^3  Mass=1  MassUnits=kg  CenterOfMass=[0 0 0]  CenterOfMassUnits=m  MomentsOfInertia=[1 1 1]  MomentsOfInertiaUnits=kg*m^2  ProductsOfInertia=[0 0 0]  ProductsOfInertiaUnits=kg*m^2  GraphicType=FromGeometry  MarkerShape=Sphere  MarkerSize=10  GraphicVisPropType=SimpleVisualProperties  GraphicDiffuseColor=[0.0 0.0 0.0]  GraphicOpacity=1  GraphicSpecularColor=[0.5 0.5 0.5 1.0]  GraphicAmbientColor=[0.15 0.15 0.15 1.0]  GraphicEmissiveColor=[0.0 0.0 0.0 1.0]  GraphicShininess=75  DoExposeReferenceFrame=off  SerializedFrames=<Frames><Frame><Id>Frame1</Id><Value><Name>F1</Name><Origin><Source>GeometricFeature</Source><FeatureName>+x -y curve</FeatureName></Origin><PrimaryAxis><DefinedDirection>+X</DefinedDirection><Source>ReferenceFrame</Source><SourceDirection>+Z</SourceDirection><FeatureName></FeatureName></PrimaryAxis><SecondaryAxis><DefinedDirection>+Y</DefinedDirection><Source>ReferenceFrame</Source><SourceDirection>+Y</SourceDirection><FeatureName></FeatureName></SecondaryAxis></Value></Frame><Frame><Id>Frame2</Id><Value><Name>F2</Name><Origin><Source>GeometricFeature</Source><FeatureName>-x -y curve</FeatureName></Origin><PrimaryAxis><DefinedDirection>+X</DefinedDirection><Source>ReferenceFrame</Source><SourceDirection>+Z</SourceDirection><FeatureName></FeatureName></PrimaryAxis><SecondaryAxis><DefinedDirection>+Y</DefinedDirection><Source>ReferenceFrame</Source><SourceDirection>+Y</SourceDirection><FeatureName></FeatureName></SecondaryAxis></Value></Frame><Frame><Id>Frame3</Id><Value><Name>C</Name><Origin><Source>GeometricFeature</Source><FeatureName>-y surface</FeatureName></Origin><PrimaryAxis><DefinedDirection>+Z</DefinedDirection><Source>ReferenceFrame</Source><SourceDirection>+Z</SourceDirection><FeatureName></FeatureName></PrimaryAxis><SecondaryAxis><DefinedDirection>+X</DefinedDirection><Source>ReferenceFrame</Source><SourceDirection>+X</SourceDirection><FeatureName></FeatureName></SecondaryAxis></Value></Frame><Frame><Id>Frame4</Id><Value><Name>F4</Name><Origin><Source>GeometricFeature</Source><FeatureName>+y surface</FeatureName></Origin><PrimaryAxis><DefinedDirection>+Z</DefinedDirection><Source>ReferenceFrame</Source><SourceDirection>+Z</SourceDirection><FeatureName></FeatureName></PrimaryAxis><SecondaryAxis><DefinedDirection>+X</DefinedDirection><Source>ReferenceFrame</Source><SourceDirection>+X</SourceDirection><FeatureName></FeatureName></SecondaryAxis></Value></Frame></Frames>
  Location : sm_lib/Frames and Transforms/Rigid Transform  RotationMethod=StandardAxis  FollAlignAxisA=+Z  BaseAlignAxisA=-Y  FollAlignAxisB=+X  BaseAlignAxisB=+X  RotationStandardAxis=+X  RotationAngle=pi/2  RotationAngleUnits=rad  RotationArbitraryAxis=[0 0 1]  RotationSequenceAxes=FollowerAxes  RotationSequence=XYX  RotationSequenceAngles=[0 0 0]  RotationSequenceAnglesUnits=deg  RotationMatrix=[1 0 0; 0 1 0; 0 0 1]  Quaternion=[1 0 0 0]  TranslationMethod=Cartesian  TranslationCartesianOffset=[0 0 4]  TranslationCartesianOffsetUnits=cm  TranslationStandardAxis=+Z  TranslationStandardOffset=0  TranslationStandardOffsetUnits=m  TranslationROffset=0  TranslationROffsetUnits=m  TranslationThetaOffset=0  TranslationThetaOffsetUnits=deg  TranslationZOffset=0  TranslationZOffsetUnits=m
  PS-Simulink Converter : nesl_utility/PS-Simulink Converter  PhysicalDomain=network_engine_domain  SubClassName=ps_output  LeftPortType=input  RightPortType=output  PseudoPeriodic=off  Frequencies=[]  VectorFormat=inherit  Unit=inherit  AffineConversion=off
  PS-Simulink Converter1 : nesl_utility/PS-Simulink Converter  PhysicalDomain=network_engine_domain  SubClassName=ps_output  LeftPortType=input  RightPortType=output  PseudoPeriodic=off  Frequencies=[]  VectorFormat=inherit  Unit=inherit  AffineConversion=off
  Planar Joint : sm_lib/Joints/Planar Joint  JointMode=Normal  CompositeWrenchDir=FollowerOnBase  CompositeWrenchFrame=BaseFrame  SenseConstraintForce=off  SenseConstraintTorque=off  SenseTotalForce=off  SenseTotalTorque=off  PxPositionTargetSpecify=off  PxPositionTargetPriority=High  PxPositionTargetValue=0  PxPositionTargetValueUnits=m  PxVelocityTargetSpecify=off  PxVelocityTargetPriority=High  PxVelocityTargetValue=0  PxVelocityTargetValueUnits=m/s  PxEquilibriumPosition=0  PxEquilibriumPositionUnits=m  PxSpringStiffness=0  PxSpringStiffnessUnits=N/m  PxDampingCoefficient=0  PxDampingCoefficientUnits=N/(m/s)  PxLowerLimitSpecify=off  PxLowerLimitBound=-1  PxLowerLimitBoundUnits=m  PxLowerLimitStiffness=1e6  PxLowerLimitStiffnessUnits=N/m  PxLowerLimitDamping=1e3  PxLowerLimitDampingUnits=N/(m/s)  PxLowerLimitTransitionRegionWidth=1e-4  PxLowerLimitTransitionRegionWidthUnits=m  PxUpperLimitSpecify=off  PxUpperLimitBound=1  PxUpperLimitBoundUnits=m  PxUpperLimitStiffness=1e6  PxUpperLimitStiffnessUnits=N/m  PxUpperLimitDamping=1e3  PxUpperLimitDampingUnits=N/(m/s)  PxUpperLimitTransitionRegionWidth=1e-4  PxUpperLimitTransitionRegionWidthUnits=m  PxTorqueActuationMode=NoTorque  PxMotionActuationMode=ComputedMotion  PxSensePosition=off  PxSenseVelocity=off  PxSenseAcceleration=off  PxSenseTorqueForce=off  PxSenseLowerLimitTorqueForce=off  PxSenseUpperLimitTorqueForce=off  PyPositionTargetSpecify=off  PyPositionTargetPriority=High  PyPositionTargetValue=0  PyPositionTargetValueUnits=m  PyVelocityTargetSpecify=off  PyVelocityTargetPriority=High  PyVelocityTargetValue=0  PyVelocityTargetValueUnits=m/s  PyEquilibriumPosition=0  PyEquilibriumPositionUnits=m  PySpringStiffness=0  PySpringStiffnessUnits=N/m  PyDampingCoefficient=0  PyDampingCoefficientUnits=N/(m/s)  PyLowerLimitSpecify=off  PyLowerLimitBound=-1  PyLowerLimitBoundUnits=m  PyLowerLimitStiffness=1e6  PyLowerLimitStiffnessUnits=N/m  PyLowerLimitDamping=1e3  PyLowerLimitDampingUnits=N/(m/s)  PyLowerLimitTransitionRegionWidth=1e-4  PyLowerLimitTransitionRegionWidthUnits=m  PyUpperLimitSpecify=off  PyUpperLimitBound=1  PyUpperLimitBoundUnits=m  PyUpperLimitStiffness=1e6  PyUpperLimitStiffnessUnits=N/m  PyUpperLimitDamping=1e3  PyUpperLimitDampingUnits=N/(m/s)  PyUpperLimitTransitionRegionWidth=1e-4  PyUpperLimitTransitionRegionWidthUnits=m  PyTorqueActuationMode=NoTorque  PyMotionActuationMode=ComputedMotion  PySensePosition=off  PySenseVelocity=off  PySenseAcceleration=off  PySenseTorqueForce=off  PySenseLowerLimitTorqueForce=off  PySenseUpperLimitTorqueForce=off  RzPositionTargetSpecify=off  RzPositionTargetPriority=High  RzPositionTargetValue=0  RzPositionTargetValueUnits=deg  RzVelocityTargetSpecify=off  RzVelocityTargetPriority=High  RzVelocityTargetValue=0  RzVelocityTargetValueUnits=deg/s  RzEquilibriumPosition=0  RzEquilibriumPositionUnits=deg  RzSpringStiffness=0  RzSpringStiffnessUnits=N*m/deg  RzDampingCoefficient=0  RzDampingCoefficientUnits=N*m/(deg/s)  RzLowerLimitSpecify=off  RzLowerLimitBound=-90  RzLowerLimitBoundUnits=deg  RzLowerLimitStiffness=1e4  RzLowerLimitStiffnessUnits=N*m/deg  RzLowerLimitDamping=10  RzLowerLimitDampingUnits=N*m/(deg/s)  RzLowerLimitTransitionRegionWidth=0.1  RzLowerLimitTransitionRegionWidthUnits=deg  RzUpperLimitSpecify=off  RzUpperLimitBound=90  RzUpperLimitBoundUnits=deg  RzUpperLimitStiffness=1e4  RzUpperLimitStiffnessUnits=N*m/deg  RzUpperLimitDamping=10  RzUpperLimitDampingUnits=N*m/(deg/s)  RzUpperLimitTransitionRegionWidth=0.1  RzUpperLimitTransitionRegionWidthUnits=deg  RzTorqueActuationMode=NoTorque  RzMotionActuationMode=ComputedMotion  RzSensePosition=off  RzSenseVelocity=off  RzSenseAcceleration=off  RzSenseTorqueForce=off  RzSenseLowerLimitTorqueForce=off  RzSenseUpperLimitTorqueForce=off
  Rate Transition1 : RateTransition  OutPortSampleTime=0.01
  Rate Transition2 : RateTransition  OutPortSampleTime=0.01
  Revolute Joint : sm_lib/Joints/Revolute Joint  JointMode=Normal  CompositeWrenchDir=FollowerOnBase  CompositeWrenchFrame=BaseFrame  SenseConstraintForce=off  SenseConstraintTorque=off  SenseTotalForce=off  SenseTotalTorque=off  PositionTargetSpecify=off  PositionTargetPriority=High  PositionTargetValue=0  PositionTargetValueUnits=deg  VelocityTargetSpecify=off  VelocityTargetPriority=High  VelocityTargetValue=0  VelocityTargetValueUnits=deg/s  EquilibriumPosition=0  EquilibriumPositionUnits=deg  SpringStiffness=0  SpringStiffnessUnits=N*m/deg  DampingCoefficient=0  DampingCoefficientUnits=N*m/(deg/s)  LowerLimitSpecify=off  LowerLimitBound=-90  LowerLimitBoundUnits=deg  LowerLimitStiffness=1e4  LowerLimitStiffnessUnits=N*m/deg  LowerLimitDamping=10  LowerLimitDampingUnits=N*m/(deg/s)  LowerLimitTransitionRegionWidth=0.1  LowerLimitTransitionRegionWidthUnits=deg  UpperLimitSpecify=off  UpperLimitBound=90  UpperLimitBoundUnits=deg  UpperLimitStiffness=1e4  UpperLimitStiffnessUnits=N*m/deg  UpperLimitDamping=10  UpperLimitDampingUnits=N*m/(deg/s)  UpperLimitTransitionRegionWidth=0.1  UpperLimitTransitionRegionWidthUnits=deg  TorqueActuationMode=NoTorque  MotionActuationMode=ComputedMotion  SensePosition=on  SenseVelocity=on  SenseAcceleration=off  SenseTorqueForce=off  SenseLowerLimitTorqueForce=off  SenseUpperLimitTorqueForce=off
  Rigid Transform : sm_lib/Frames and Transforms/Rigid Transform  RotationMethod=StandardAxis  FollAlignAxisA=+X  BaseAlignAxisA=+Y  FollAlignAxisB=+Y  BaseAlignAxisB=+Z  RotationStandardAxis=+Y  RotationAngle=-90  RotationAngleUnits=deg  RotationArbitraryAxis=[0 0 1]  RotationSequenceAxes=FollowerAxes  RotationSequence=XYX  RotationSequenceAngles=[0 0 0]  RotationSequenceAnglesUnits=deg  RotationMatrix=[1 0 0;0 1 0;0 0 1]  Quaternion=[1 0 0 0]  TranslationMethod=None  TranslationCartesianOffset=[0 0 0]  TranslationCartesianOffsetUnits=m  TranslationStandardAxis=+Z  TranslationStandardOffset=0  TranslationStandardOffsetUnits=m  TranslationROffset=0  TranslationROffsetUnits=m  TranslationThetaOffset=0  TranslationThetaOffsetUnits=deg  TranslationZOffset=0  TranslationZOffsetUnits=m
  Rigid Transform1 : sm_lib/Frames and Transforms/Rigid Transform  RotationMethod=StandardAxis  FollAlignAxisA=+X  BaseAlignAxisA=+Y  FollAlignAxisB=+Y  BaseAlignAxisB=+Z  RotationStandardAxis=+Y  RotationAngle=90  RotationAngleUnits=deg  RotationArbitraryAxis=[0 0 1]  RotationSequenceAxes=FollowerAxes  RotationSequence=XYX  RotationSequenceAngles=[0 0 0]  RotationSequenceAnglesUnits=deg  RotationMatrix=[1 0 0;0 1 0;0 0 1]  Quaternion=[1 0 0 0]  TranslationMethod=None  TranslationCartesianOffset=[0 0 0]  TranslationCartesianOffsetUnits=m  TranslationStandardAxis=+Z  TranslationStandardOffset=0  TranslationStandardOffsetUnits=m  TranslationROffset=0  TranslationROffsetUnits=m  TranslationThetaOffset=0  TranslationThetaOffsetUnits=deg  TranslationZOffset=0  TranslationZOffsetUnits=m
  Spatial Contact Force3 : sm_lib/Forces and Torques/Spatial Contact Force  SenseSeparationDistance=off  NormalForceType=SmoothSpringDamper  NormalStiffness=1e6  NormalStiffnessUnits=N/m  NormalDamping=1e3  NormalDampingUnits=N/(m/s)  NormalTransitionRegionWidth=1e-4  NormalTransitionRegionWidthUnits=m  FrictionType=None  CoefficientOfStaticFriction=0.3  CoefficientOfDynamicFriction=0.3  FrictionalCriticalVelocity=0.2  FrictionalCriticalVelocityUnits=m/s  SenseContactSignal=off  SensePenetrationDepth=off  SenseNormalVelocity=off  SenseTangentialVelocity=off  SensingForceTorqueDirection=BaseOnFollower  SensingForceTorqueResolutionFrame=ContactFrame  SenseNormalForce=off  SenseNormalForceMagnitude=off  SenseNormalTorque=off  SenseFrictionalForce=off  SenseFrictionalForceMagnitude=off  SenseFrictionalTorque=off  SenseTotalForce=off  SenseTotalTorque=off  SenseContactBaseRotation=off  SenseContactBaseTranslation=off  SenseContactFollowerRotation=off  SenseContactFollowerTranslation=off  ZeroCrossDetectContactStartAndEnd=off
  Spatial Contact Force4 : sm_lib/Forces and Torques/Spatial Contact Force  SenseSeparationDistance=off  NormalForceType=SmoothSpringDamper  NormalStiffness=1e6  NormalStiffnessUnits=N/m  NormalDamping=1e3  NormalDampingUnits=N/(m/s)  NormalTransitionRegionWidth=1e-4  NormalTransitionRegionWidthUnits=m  FrictionType=None  CoefficientOfStaticFriction=0.3  CoefficientOfDynamicFriction=0.3  FrictionalCriticalVelocity=0.2  FrictionalCriticalVelocityUnits=m/s  SenseContactSignal=off  SensePenetrationDepth=off  SenseNormalVelocity=off  SenseTangentialVelocity=off  SensingForceTorqueDirection=BaseOnFollower  SensingForceTorqueResolutionFrame=ContactFrame  SenseNormalForce=off  SenseNormalForceMagnitude=off  SenseNormalTorque=off  SenseFrictionalForce=off  SenseFrictionalForceMagnitude=off  SenseFrictionalTorque=off  SenseTotalForce=off  SenseTotalTorque=off  SenseContactBaseRotation=off  SenseContactBaseTranslation=off  SenseContactFollowerRotation=off  SenseContactFollowerTranslation=off  ZeroCrossDetectContactStartAndEnd=off
  Wheel1 : PMIOPort  Side=Left
  BumperContact : PMIOPort  Port=2  Side=Left
  Wheel2 : PMIOPort  Port=3  Side=Right
  World : PMIOPort  Port=4  Side=Right
  Ref : PMIOPort  Port=5  Side=Right
  angles : Outport
  omega_x : Outport  Port=2
  wires:
  PS-Simulink Converter/1 -> Rate Transition1/1
  PS-Simulink Converter1/1 -> Rate Transition2/1
  Rate Transition2/1 -> omega_x/1
  Rate Transition1/1 -> angles/1
  connections:
  World/RConn1 -- Planar Joint/LConn1
  Revolute Joint/LConn1 -- Rigid Transform/RConn1
  Wheel1/RConn1 -- Case_main/LConn1
  Case_main/RConn1 -- Wheel2/RConn1
  CAD_Body/RConn1 -- Case_main/LConn2 -- Rigid Transform1/RConn1 -- Ref/RConn1
  Spatial Contact Force3/LConn1 -- BumperContact/RConn1 -- Spatial Contact Force4/LConn1
  Spatial Contact Force3/RConn1 -- CAD_Bumper/RConn2
  Spatial Contact Force4/RConn1 -- CAD_Bumper/RConn1
  Case_main/RConn2 -- CAD_Bumper/LConn1
  Revolute Joint/RConn2 -- PS-Simulink Converter/LConn1
  Revolute Joint/RConn3 -- PS-Simulink Converter1/LConn1
  Planar Joint/RConn1 -- Location/LConn1
  Rigid Transform/LConn1 -- Location/RConn1
  Rigid Transform1/LConn1 -- Revolute Joint/RConn1
